simulink model "ben3asys"  (Simulink 6.0)
settings: Solver=ode23  SolverMode=SingleTasking  StartTime=0.0  StopTime=4  RelTol=1e-3  AbsTol=1e-6
PreLoadFcn:
  | ben3adat
values from neighbouring files (symbols this model uses):
  gd1 = 1    [ben2bdat.m]    (also in ben2cdat.m = [1/950,1]; ben3bdat.m = [1,6,13])
  gd3 = [1/85/85,1.2/85,1]    [ben2bdat.m]    (also in ben2cdat.m; ben3bdat.m = [1,-1])
  gd4 = 1    [ben2bdat.m]    (also in ben2cdat.m = [1/775/775,1/775,1]; ben3bdat.m = [1,-0.6667])
  gd5 = [1/170,1]    [ben2bdat.m]    (also in ben2cdat.m; ben3bdat.m = [1,-1])
  gd6 = [1,-0.6873]    [ben3bdat.m]
  gd7 = [1,0]    [ben2bdat.m]    (also in ben2cdat.m; ben3bdat.m = [1,-0.9277])
  gn1_gn2 = [gn1;gn2]    [ben3bdat.m]
  gn3 = 1    [ben2bdat.m]    (also in ben2cdat.m; ben3bdat.m = .2625*[1,-0.9048])
  gn4 = 1    [ben2bdat.m]    (also in ben2cdat.m; ben3bdat.m = 1.7*[1,-0.9608])
  gn5 = 1    [ben2bdat.m]    (also in ben2cdat.m; ben3bdat.m = 1.035*[1,-0.9324])
  gn6 = 0.1564*[1,1]    [ben3bdat.m]
  gn7 = 1    [ben2bdat.m]    (also in ben2cdat.m; ben3bdat.m = 0.0362*[1,1])
  offT1 = 1.0e-8    (= 1e-08)    [ben3bdat.m]
  offT2 = 0.0    (= 0)    [ben3bdat.m]
  offZOH = 2.0e-8    (= 2e-08)    [ben3bdat.m]
  T1 = 1/50    (= 0.02)    [ben3bdat.m]
  T2 = 1/200    (= 0.005)    [ben3bdat.m]
settings Model: Creator=The MathWorks Inc.  LastModifiedBy=batserve  ExtModeTrigMode=oneshot  ExtModeArmWhenConnect=off  ExtModeAutoUpdateStatusClock=off
settings DataIOCC: ExternalInput=[]  InitialState=[]  LimitDataPoints=off  SaveOutput=off  SaveTime=off
settings OptimizationCC: BooleanDataType=off
settings DebuggingCC: CheckExecutionContextPreStartOutputMsg=on  CheckExecutionContextRuntimeOutputMsg=on  SolverPrmCheckMsg=none  IntegerOverflowMsg=none
settings HardwareCC: TargetUnknown=on

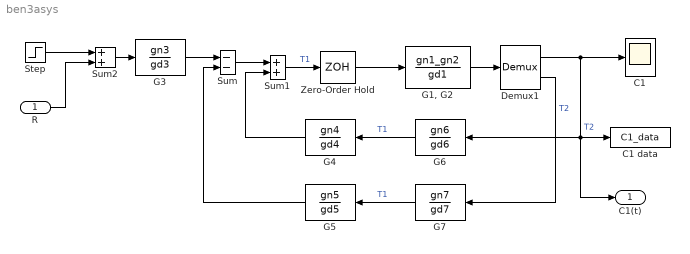
== system ben3asys ==
  R : Inport  Port=1  LatchInput=off
  C1 : Scope
      settings: TickLabels=on  YMin=0  YMax=1.4  DataFormat=Array
  C1 data : ToWorkspace  VariableName=C1_data  SampleTime=-1  SaveFormat=Array
      settings: MaxDataPoints=12000
  Demux1 : Demux  Outputs=2
  "G1, G2" : TransferFcn  Numerator=gn1_gn2  Denominator=gd1
  G3 : DiscreteTransferFcn  Numerator=gn3  Denominator=gd3  SampleTime=[T1,offT1]
  G4 : DiscreteTransferFcn  Orientation=left  Numerator=gn4  Denominator=gd4  SampleTime=[T1,offT1]
  G5 : DiscreteTransferFcn  Orientation=left  Numerator=gn5  Denominator=gd5  SampleTime=[T1,offT1]
  G6 : DiscreteTransferFcn  Orientation=left  Numerator=gn6  Denominator=gd6  SampleTime=[T2,offT2]
  G7 : DiscreteTransferFcn  Orientation=left  Numerator=gn7  Denominator=gd7  SampleTime=[T2,offT2]
  Step : Step  Time=0  SampleTime=0
  Sum : Sum  Inputs=--  SaturateOnIntegerOverflow=on  InputSameDT=on
  Sum1 : Sum  Inputs=2  SaturateOnIntegerOverflow=on  InputSameDT=on
  Sum2 : Sum  SaturateOnIntegerOverflow=on  InputSameDT=on
  Zero-Order Hold : ZeroOrderHold  SampleTime=[T1,offZOH]
  C1(t) : Outport  InitialOutput=0
  wires:
  Demux1/1 -> C1/1, C1(t)/1, C1 data/1, G6/1  "T2"
  Demux1/2 -> G7/1  "T2"
  "G1, G2"/1 -> Demux1/1
  Zero-Order Hold/1 -> "G1, G2"/1
  G7/1 -> G5/1  "T1"
  Sum/1 -> Sum1/1
  Sum1/1 -> Zero-Order Hold/1  "T1"
  G3/1 -> Sum/1
  G6/1 -> G4/1  "T1"
  G4/1 -> Sum1/2
  G5/1 -> Sum/2
  Step/1 -> Sum2/1
  R/1 -> Sum2/2
  Sum2/1 -> G3/1
